simulink model "ev_traction_simulink_model"  (R2023b)
settings: Solver=VariableStepAuto  StartTime=0.0  StopTime=10.0  RelTol=1e-3
values from neighbouring files (symbols this model uses):
  g = 9.81    [ev_traction_simulation.m]
  k = 0.3    [ev_traction_simulation.m]
  Kp = 650    [ev_traction_simulation.m]
  Kt = 0.5    [ev_traction_simulation.m]
  m = 1000    [ev_traction_simulation.m]
  r = 0.3    [ev_traction_simulation.m]
  v_ref = 20    [ev_traction_simulation.m]
settings Model: Creator=lenovo  LastModifiedBy=lenovo

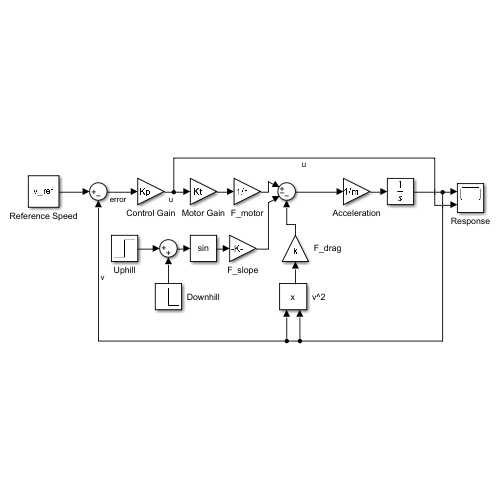
[thumbnail: Simulink's stored preview of the top-level diagram]
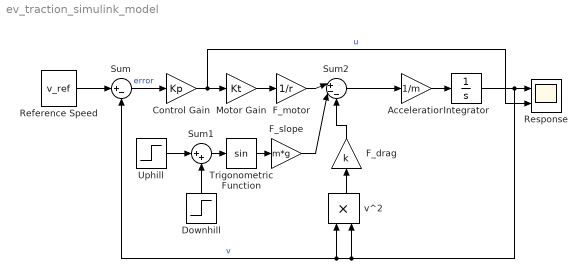
== system ev_traction_simulink_model ==
  Acceleration : Gain  Gain=1/m
  Control Gain : Gain  Gain=Kp
  Downhill : Step  Time=8  After=-5*pi/180  SampleTime=0
  F_drag : Gain  Gain=k
  F_motor : Gain  Gain=1/r
  F_slope : Gain  Gain=m*g
  Integrator : Integrator
  Motor Gain : Gain  Gain=Kt
  Reference Speed : Constant  Value=v_ref
  Response : Scope  NumInputPorts=2
  Sum : Sum  Inputs=|+-
  Sum1 : Sum  Inputs=|++
  Sum2 : Sum  Inputs=|+--
  Trigonometric Function : Trigonometry
  Uphill : Step  Time=5  After=5*pi/180  SampleTime=0
  v^2 : Product
  wires:
  Reference Speed/1 -> Sum/1
  Sum/1 -> Control Gain/1  "error"
  Control Gain/1 -> Response/2, Motor Gain/1  "u"
  Motor Gain/1 -> F_motor/1
  F_motor/1 -> Sum2/1
  Sum2/1 -> Acceleration/1
  Acceleration/1 -> Integrator/1
  Integrator/1 -> Response/1, v^2/2, v^2/1, Sum/2  "v"
  F_drag/1 -> Sum2/3
  v^2/1 -> F_drag/1
  Uphill/1 -> Sum1/1
  Trigonometric Function/1 -> F_slope/1
  Sum1/1 -> Trigonometric Function/1
  F_slope/1 -> Sum2/2
  Downhill/1 -> Sum1/2
